simulink model "dc_motor_open_loop.slx"  (R2023b)
settings: Solver=VariableStepAuto  StartTime=0.0  StopTime=20  RelTol=1e-3
settings Model: Creator=Ali  LastModifiedBy=Ali

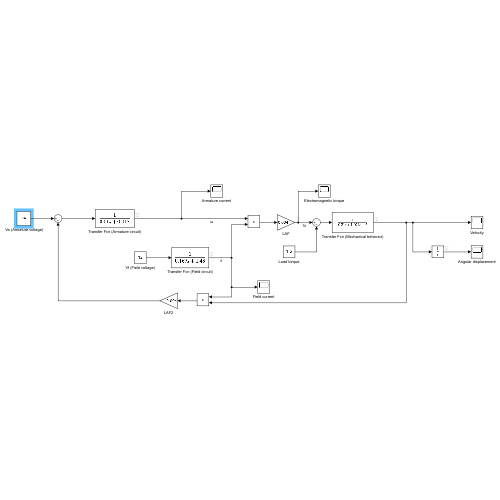
[thumbnail: Simulink's stored preview of the top-level diagram]
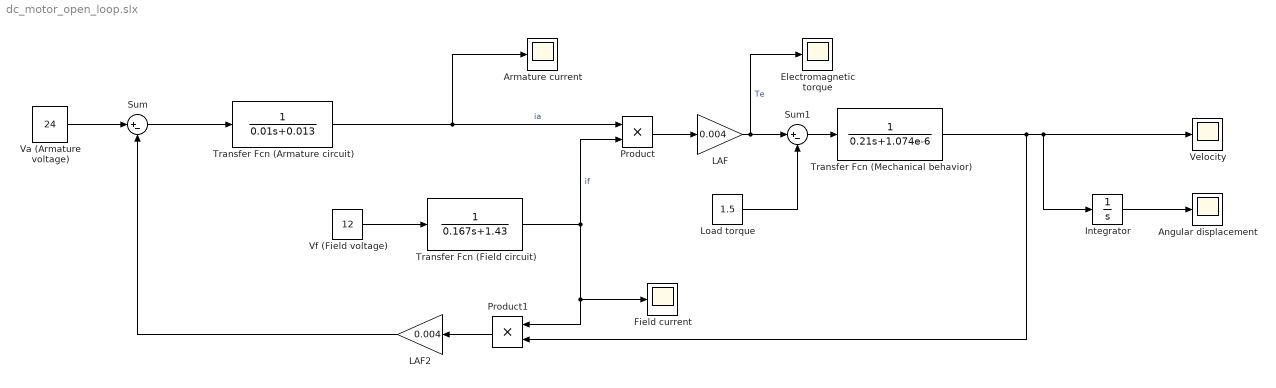
== system dc_motor_open_loop.slx ==
  " Va (Armature voltage)" : Constant  Value=24
  Angular displacement : Scope
  Armature current : Scope
  Electromagnetic torque : Scope
  Field current : Scope
  Integrator : Integrator
  LAF : Gain  Gain=0.004
  LAF2 : Gain  Gain=0.004
  Load torque : Constant  Value=1.5
  Product : Product
  Product1 : Product
  Sum : Sum  Inputs=|+-
  Sum1 : Sum  Inputs=|+-
  Transfer Fcn (Armature circuit) : TransferFcn  Denominator=[0.01 0.013]
  Transfer Fcn (Field circuit) : TransferFcn  Denominator=[0.167 1.43]
  Transfer Fcn (Mechanical behavior) : TransferFcn  Denominator=[0.21 1.074e-6]
  Velocity : Scope
  Vf (Field voltage) : Constant  Value=12
  wires:
  " Va (Armature voltage)"/1 -> Sum/1
  LAF2/1 -> Sum/2
  Sum/1 -> Transfer Fcn (Armature circuit)/1
  Transfer Fcn (Armature circuit)/1 -> Armature current/1, Product/1  "ia"
  Vf (Field voltage)/1 -> Transfer Fcn (Field circuit)/1
  Transfer Fcn (Field circuit)/1 -> Field current/1, Product1/1, Product/2  "if"
  Product/1 -> LAF/1
  LAF/1 -> Electromagnetic torque/1, Sum1/1  "Te"
  Load torque/1 -> Sum1/2
  Sum1/1 -> Transfer Fcn (Mechanical behavior)/1
  Transfer Fcn (Mechanical behavior)/1 -> Product1/2, Integrator/1, Velocity/1
  Integrator/1 -> Angular displacement/1
  Product1/1 -> LAF2/1
